simulink model "SimulinkMaskTest"  (R2023a)
settings: Solver=FixedStepDiscrete  StartTime=0.0  StopTime=10  FixedStep=0.002  RelTol=1e-3  EnableMultiTasking=on
model workspace (MAT data in the model file):
  gain = 0.25
libraries: simulink x3, hdlsllib x1
settings Model: ExtModeTrigDuration=10000  Creator=auw_a  LastModifiedBy=auw_a
settings SolverCC: AlgebraicLoopSolver=TrustRegion  PositivePriorityOrder=on
settings DataIOCC: ExternalInput=[t', a', b']  LoadExternalInput=on  ReturnWorkspaceOutputs=off
settings OptimizationCC: LifeSpan=inf
settings DebuggingCC: UnconnectedInputMsg=warning  UnconnectedOutputMsg=warning  UnconnectedLineMsg=warning  ArithmeticOperatorsInVariantConditions=warning
settings ModelReferenceCC: EnableRefExpFcnMdlSchedulingChecks=on
settings SFSimCC: SimUseLocalCustomCode=off  CustomCodeUndefinedFunction=UseInterfaceOnly
settings RTWCC: Description=QUARC Win64 Target  SystemTargetFile=quarc_win64.tlc  TemplateMakefile=quarc_default_tmf  RTWUseLocalCustomCode=off
settings CodeAppCC: StateflowObjectComments=on
settings STFCustomTargetCC: TargetPreCompLibLocation=C:\PROGRA~3\QUARC\lib\2016a\win64\release  UseToolchainInfoCompliant=off  SystemTargetFile=quarc_win64.tlc
settings GRTTargetCC: TargetPreCompLibLocation=C:\PROGRA~3\QUARC\lib\2016a\win64\release  ParMdlRefBuildCompliant=off  CompOptLevelCompliant=off  CombineOutputUpdateFcns=off  MatFileLogging=off  CPPClassGenCompliant=off  GRTInterface=on  UseToolchainInfoCompliant=off  ExtMode=on  ExtModeMexFile=quarc_comm
settings ConfigComp: CovMetricSettings=dswe

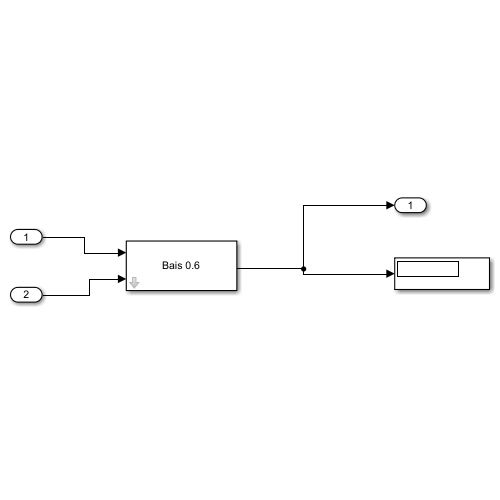
[thumbnail: Simulink's stored preview of the top-level diagram]
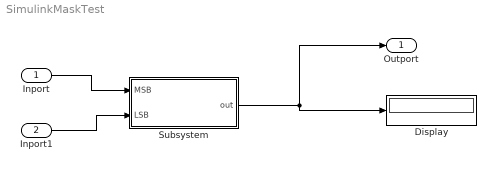
== system SimulinkMaskTest ==
  Inport : Inport  OutDataTypeStr=double  PortDimensions=1
  Inport1 : Inport  Port=2  OutDataTypeStr=double  PortDimensions=1
  Display : Display
  Subsystem : Subsystem  mask{gain=.6}
      mask prompts: gain "Enter Bais Value"
      mask init:
      | str = "Bais " + gain;
      | label = str;
      mask Display: disp(label);
  Outport : Outport  PortDimensions=1
  wires:
  Subsystem/1(out) -> Display/1, Outport/1
  Inport/1 -> Subsystem/1(MSB)
  Inport1/1 -> Subsystem/2(LSB)

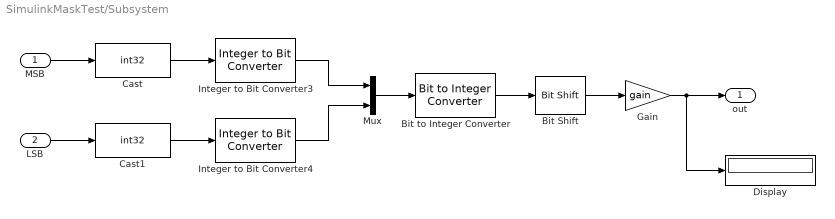
== system SimulinkMaskTest/Subsystem ==
  MSB : Inport
  LSB : Inport  Port=2
  Bit Shift : hdlsllib/Logic and Bit Operations/Bit Shift  mode=Shift Right Logical  N=3
  Bit to Integer Converter : simulink/Logic and Bit Operations/Bit to Integer Converter  nbits=16  bitOrder=MSB first  signedOutputValues=Unsigned  outDtype=Inherit via internal rule  outDtypeSigned=Inherit via internal rule
  Cast : DataTypeConversion  OutDataTypeStr=int32  SaturateOnIntegerOverflow=off  RndMeth=Floor
  Cast1 : DataTypeConversion  OutDataTypeStr=int32  SaturateOnIntegerOverflow=off  RndMeth=Floor
  Display : Display
  Gain : Gain  Gain=gain
  Integer to Bit Converter3 : simulink/Logic and Bit Operations/Integer to Bit Converter  nbits=8  signedInputValues=Unsigned  bitOrder=MSB first  outDtype=Same as input
  Integer to Bit Converter4 : simulink/Logic and Bit Operations/Integer to Bit Converter  nbits=8  signedInputValues=Unsigned  bitOrder=MSB first  outDtype=Same as input
  Mux : Mux  Inputs=2
  out : Outport
  wires:
  Integer to Bit Converter4/1 -> Mux/2
  Bit to Integer Converter/1 -> Bit Shift/1
  Bit Shift/1 -> Gain/1
  Integer to Bit Converter3/1 -> Mux/1
  Mux/1 -> Bit to Integer Converter/1
  Gain/1 -> Display/1, out/1
  MSB/1 -> Cast/1
  Cast/1 -> Integer to Bit Converter3/1
  Cast1/1 -> Integer to Bit Converter4/1
  LSB/1 -> Cast1/1
